simulink model "Lab12sym"  (R2021b)
settings: Solver=VariableStepAuto  StartTime=0.0  StopTime=10.0  RelTol=1e-3
values from neighbouring files (symbols this model uses):
  a0 = 1    [Lab12.m]
  a1 = -(3*T+2)    (= -2.3)    [Lab12.m]
  a2 = (1+2*T)*(1+T)    (= 1.32)    [Lab12.m]
  b2 = 3*T^2    (= 0.03)    [Lab12.m]
  T = 0.1    [Lab12.m]
undefined symbols (not defined in the file or in its folder): P, R, Rinf
settings Model: Creator=fabian  LastModifiedBy=fabian

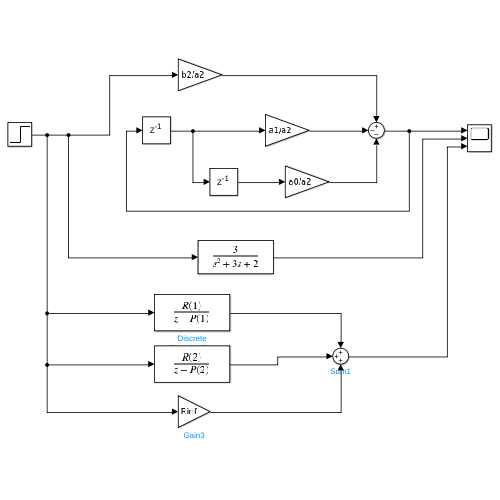
[thumbnail: Simulink's stored preview of the top-level diagram]
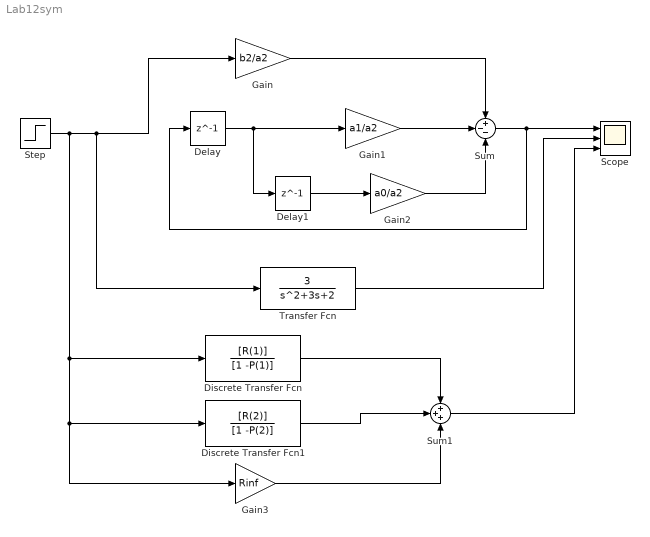
== system Lab12sym ==
  Delay : Delay  DelayLength=1  SampleTime=T
  Delay1 : Delay  DelayLength=1  SampleTime=T
  Discrete Transfer Fcn : DiscreteTransferFcn  Numerator=[R(1)]  Denominator=[1 -P(1)]
  Discrete Transfer Fcn1 : DiscreteTransferFcn  Numerator=[R(2)]  Denominator=[1 -P(2)]
  Gain : Gain  Gain=b2/a2
  Gain1 : Gain  Gain=a1/a2
  Gain2 : Gain  Gain=a0/a2
  Gain3 : Gain  Gain=Rinf
  Scope : Scope  NumInputPorts=3
  Step : Step  Time=0  SampleTime=0
  Sum : Sum  Inputs=+--
  Sum1 : Sum  Inputs=+++
  Transfer Fcn : TransferFcn  Numerator=[3]  Denominator=[1 3 2]
  wires:
  Step/1 -> Discrete Transfer Fcn/1, Discrete Transfer Fcn1/1, Gain3/1, Transfer Fcn/1, Gain/1
  Gain/1 -> Sum/1
  Sum/1 -> Scope/1, Delay/1
  Delay/1 -> Delay1/1, Gain1/1
  Gain1/1 -> Sum/2
  Gain2/1 -> Sum/3
  Delay1/1 -> Gain2/1
  Transfer Fcn/1 -> Scope/2
  Discrete Transfer Fcn/1 -> Sum1/1
  Discrete Transfer Fcn1/1 -> Sum1/2
  Gain3/1 -> Sum1/3
  Sum1/1 -> Scope/3
